simulink model "driver_model"  (R2024b)
settings: Solver=FixedStepAuto  StartTime=0.0  StopTime=10.0  FixedStep=Ts  RelTol=1e-3
values from neighbouring files (symbols this model uses):
  lapData = table(distance, vitesse, x, y, aYaw)    [trackdata_extended.m]    (also in trackdata_skidpad.m)
undefined symbols (not defined in the file or in its folder): DiscIntNeverNeededParam, lr, m
libraries: simulink x2, vehdynlibdriver x1, autolibshared x1
settings Model: Creator=marti  LastModifiedBy=marti

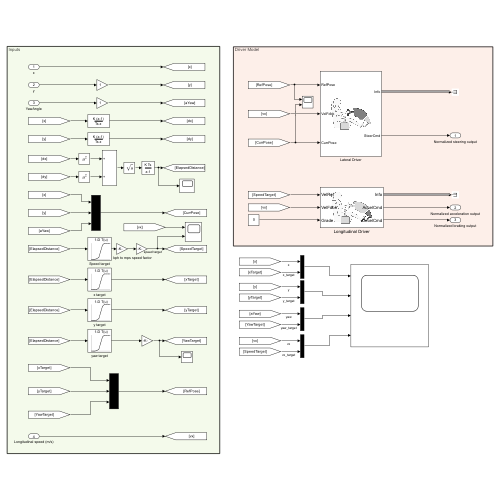
[thumbnail: Simulink's stored preview of the top-level diagram]
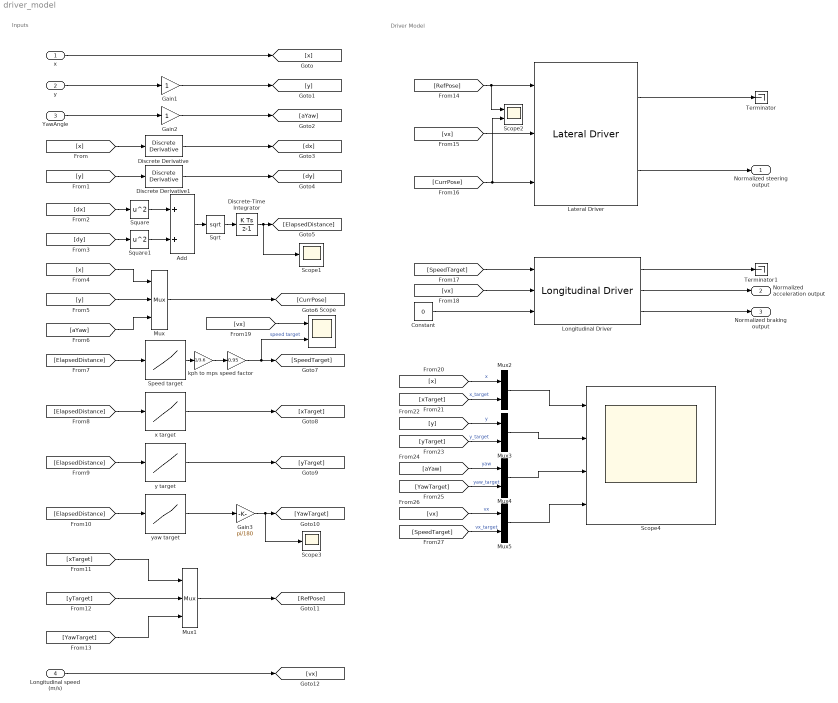
== system driver_model ==
  note: Driver Model
  note: Inputs
  x : Inport
  y : Inport  Port=2
  YawAngle : Inport  Port=3
  Longitudinal speed (m/s) : Inport  Port=4
  Add : Sum
  Constant : Constant  Value=0
  Discrete Derivative : simulink/Discrete/Discrete Derivative  gainval=1.0  ICPrevScaledInput=0.0  OutMin=[]  OutMax=[]  OutDataType=fixdt(1, 16)  OutScaling=2^-10  DoSatur=off
  Discrete Derivative1 : simulink/Discrete/Discrete Derivative  gainval=1.0  ICPrevScaledInput=0.0  OutMin=[]  OutMax=[]  OutDataType=fixdt(1, 16)  OutScaling=2^-10  DoSatur=off
  Discrete-Time Integrator : DiscreteIntegrator  SampleTime=-1  ICPrevOutput=DiscIntNeverNeededParam  ICPrevScaledInput=DiscIntNeverNeededParam
  Gain1 : Gain
  Gain2 : Gain
  Gain3 : Gain  Gain=pi/180
  Lateral Driver : vehdynlibdriver/Lateral Driver  extSteerOvr=off  extSteerHld=off  extSteerZero=off  steerOut=off  cntrlTypeLat=Stanley  coordMode=SAE J670 (Z-down)  angUnits=rad  tau=0.1  L=3  vecPose=on  dynamMode=off  PositionGainF=2.5  PositionGainR=2.5  YawRateGain=.2  DelayGain=.2  a=lf  b=lr  m=2016  Cy_f=25266  Cy_r=70933  I=4013  Ksteer=18  theta=30*pi/180  aMode=2
  Longitudinal Driver : autolibshared/Longitudinal Driver  extAccelOvr=off  extDecelOvr=off  extAccelHld=off  extDecelHld=off  extAccelZero=off  extDecelZero=off  cntrlType=PI  shftType=None  velUnits=m/s  gearOut=off  Kp=4  Ki=0.5  Kff=.1  Kg=0  VehVelVec=[0 100]  KffVec=[.1 .1]  KpVec=[10 10]  KiVec=[5 5]  KgVec=[0 0]  m=m  Kpt=3000  tau=.1  L=2  aR=200  bR=2.5  cR=.5  g=9.81  vnom=10  Kaw=1  tauerr=.01  tauPt=2  GearInit=0  tShift=.1  pdlVec=[0.1 0.4 0.5 0.9]  upShftTbl=[-1 12.9375 26.4375 39.9375 51.18749999999999 62.4375 72.84375 83.25;-1 16.3125 29.8125 43.3125 54.5624 65.8125 76.78125 87.75;-1 19.6875 33.1875 46.68749999999999 57.9375 69.1875 80.71875 92.25;-1 33 52.5 77.25 100.5 138.75 161.875 185]  dwnShftTbl=[1 9.5625 23.0625 36.5625 47.8125 59.0625 68.90625 78.75;1 12.9375 26.4375 39.9375 51.18749999999999 62.4375 72.84375 83.25;1 16.3125 29.8125 43.3125 54.562499 65.8125 76.78125 87.75;1 19.6875 33.1875 46.68749999999999 57.9375 69.1875 80.71875 92.25]  tClutch=.5  tRev=.5  tPark=120  aMode=2  UpGearVec="[0  1  2  3  4  5  6  7]"  DownGearVec="[1  2  3  4  5  6  7  8]"
      settings: LibrarySourceBlock=vehdynlibdriver/Longitudinal Driver
  Mux : Mux  Inputs=3
  Mux1 : Mux  Inputs=3
  Mux{2..5} (4 alike) : Mux  Inputs=2
  Scope : Scope  NumInputPorts=2
  Scope1 : Scope
  Scope2 : Scope  NumInputPorts=2
  Scope3 : Scope
  Scope4 : Scope  NumInputPorts=4
  Speed target : Lookup_n-D  NumberOfTableDimensions=1  BreakpointsForDimension1=lapData.distance  Table=lapData.vitesse  InternalRulePriority=Speed  RndMeth=Simplest
  Sqrt : Sqrt
  Square : Math  Operator=square
  Square1 : Math  Operator=square
  Terminator : Terminator
  Terminator1 : Terminator
  kph to mps : Gain  Gain=1/3.6
  speed factor : Gain  Gain=0.95
  x target : Lookup_n-D  NumberOfTableDimensions=1  BreakpointsForDimension1=lapData.distance  Table=lapData.x  InternalRulePriority=Speed  RndMeth=Simplest
  y target : Lookup_n-D  NumberOfTableDimensions=1  BreakpointsForDimension1=lapData.distance  Table=lapData.y  InternalRulePriority=Speed  RndMeth=Simplest
  yaw target : Lookup_n-D  NumberOfTableDimensions=1  BreakpointsForDimension1=lapData.distance  Table=lapData.aYaw  InternalRulePriority=Speed  RndMeth=Simplest
  Normalized steering output : Outport
  Normalized acceleration output : Outport  Port=2
  Normalized braking output : Outport  Port=3
  wires:
  x/1 -> [x]
  y/1 -> Gain1/1
  YawAngle/1 -> Gain2/1
  [x] -> Discrete Derivative/1
  [y] -> Discrete Derivative1/1
  Discrete Derivative/1 -> [dx]
  Discrete Derivative1/1 -> [dy]
  [dx] -> Square/1
  [dy] -> Square1/1
  Square/1 -> Add/1
  Square1/1 -> Add/2
  Add/1 -> Sqrt/1
  Sqrt/1 -> Discrete-Time Integrator/1
  [y] -> Mux/2
  [x] -> Mux/1
  [aYaw] -> Mux/3
  Mux/1 -> [CurrPose]
  [ElapsedDistance] -> Speed target/1
  Speed target/1 -> kph to mps/1
  x target/1 -> [xTarget]
  [ElapsedDistance] -> x target/1
  [ElapsedDistance] -> y target/1
  y target/1 -> [yTarget]
  yaw target/1 -> Gain3/1
  [ElapsedDistance] -> yaw target/1
  [yTarget] -> Mux1/2
  [xTarget] -> Mux1/1
  [YawTarget] -> Mux1/3
  Mux1/1 -> [RefPose]
  Longitudinal speed (m/s)/1 -> [vx]
  [RefPose] -> Scope2/1, Lateral Driver/1
  [vx] -> Lateral Driver/2
  [CurrPose] -> Scope2/2, Lateral Driver/3
  [vx] -> Longitudinal Driver/2
  Constant/1 -> Longitudinal Driver/3
  Lateral Driver/1 -> Terminator/1
  Longitudinal Driver/1 -> Terminator1/1
  Lateral Driver/2 -> Normalized steering output/1
  Longitudinal Driver/2 -> Normalized acceleration output/1
  Longitudinal Driver/3 -> Normalized braking output/1
  [vx] -> Scope/1
  kph to mps/1 -> speed factor/1
  Gain1/1 -> [y]
  Gain2/1 -> [aYaw]
  Discrete-Time Integrator/1 -> Scope1/1, [ElapsedDistance]
  Gain3/1 -> Scope3/1, [YawTarget]
  [SpeedTarget] -> Longitudinal Driver/1
  [x] -> Mux2/1  "x"
  [xTarget] -> Mux2/2  "x_target"
  [y] -> Mux3/1  "y"
  [yTarget] -> Mux3/2  "y_target"
  [aYaw] -> Mux4/1  "yaw"
  [YawTarget] -> Mux4/2  "yaw_target"
  [vx] -> Mux5/1  "vx"
  [SpeedTarget] -> Mux5/2  "vx_target"
  Mux2/1 -> Scope4/1
  Mux3/1 -> Scope4/2
  Mux4/1 -> Scope4/3
  Mux5/1 -> Scope4/4
  speed factor/1 -> Scope/2, [SpeedTarget]  "speed target"
